simulink model "Vehicle_Model_Track_contABS"  (R2022b)
settings: Solver=ode2  StartTime=T0  StopTime=Tf  FixedStep=Ts  EnableMultiTasking=on
model workspace (MAT data in the model file):
  aKalman : Simulink.Parameter (value not decoded)
  slipEnabler : Simulink.Parameter (value not decoded)
values from neighbouring files (symbols this model uses):
  enable_onlinePlots = 0    [mainVehicleModel_2Track_contABS.m]
  enable_zoom = 1    [mainVehicleModel_2Track_contABS.m]
  hv = 0.2    [mainVehicleModel_2Track_contABS.m]
  lambda1_th = 0.1    [mainVehicleModel_2Track_contABS.m]
  lambda2_th = 0.1    [mainVehicleModel_2Track_contABS.m]
  LLC_sampleTime = LLC.sample_time    [mainVehicleModel_2Track_contABS.m]
  longCTRparam = longitController()    [mainVehicleModel_2Track_contABS.m]
  low_level_control = scenario_data.vehicle_control.low_level_control    [mainVehicleModel_2Track_contABS.m]
  omega_LPF = 100    [mainVehicleModel_2Track_contABS.m]
  previewPointParams = previewPointControllerParams()    [mainVehicleModel_2Track_contABS.m]
  rho = 0.97    [mainVehicleModel_2Track_contABS.m]
  rho_off = 0.9    [mainVehicleModel_2Track_contABS.m]
  rho_on = 1.02    [mainVehicleModel_2Track_contABS.m]
  road_data_sampled = [scenario_data.path.x_sampled', scenario_data.path.y_sampled']    [mainVehicleModel_2Track_contABS.m]
  T0 = scenario_data.times.t0    [mainVehicleModel_2Track_contABS.m]
  tau_delta = vehicle_data.steering_system.tau_D    [mainVehicleModel_2Track_contABS.m]
  Tb_dot_max = 5e3    (= 5000)    [mainVehicleModel_2Track_contABS.m]
  Tb_max = 3500    [mainVehicleModel_2Track_contABS.m]
  Tf = scenario_data.times.tf    [mainVehicleModel_2Track_contABS.m]
  Ts = scenario_data.times.step_size    [mainVehicleModel_2Track_contABS.m]
  v_on = 2.5    [mainVehicleModel_2Track_contABS.m]
  v_stop = 0.1    [mainVehicleModel_2Track_contABS.m]
  vehicle_data = getVehicleDataStruct()    [mainVehicleModel_2Track_contABS.m]
  X0 = loadInitialConditions(scenario_data.vehicle_control.max_speed/3.6)    [mainVehicleModel_2Track_contABS.m]
undefined symbols (not defined in the file or in its folder): DiscIntNeverNeededParam, latContr_select
libraries: simulink_extras x20, simulink x9, dspsigops x4, drivingvehiclecontroller x2
(part 2 of 2)

== matlab function Vehicle_Model_Track_contABS/ABS and Wheel torque generation/ABS Rear Right Wheel/compute lambda ==
  data: u input; lambda output; omega input; vehicle_data parameter
function lambda = compute_lambda(u, omega, vehicle_data)

lambda = (u - omega*vehicle_data.rear_wheel.Rr)/u;

== matlab function Vehicle_Model_Track_contABS/Vehicle Model ==
  settings: sampleTime=step_size
  data: dX_prev input; X input; Tw__rr_brake input; Tw__rl_brake input; Tw__fr_brake input; Tw__fl_brake input; Tm_req input; dX output; extra_params output; delta_req input; vehicle_data parameter; road_condition input
function [dX,extra_params] = Vehicle_model(dX_prev,X,Tw__rr_brake,Tw__rl_brake,Tw__fr_brake,Tw__fl_brake,Tm_req,delta_req,vehicle_data,road_condition)

% ----------------------------------------------------------------
%% Double Track Vehicle Model
%  authors: 
%  rev. 1.0 Mattia Piccinini & Gastone Pietro Papini Rosati
%  rev. 2.0 Edoardo Pagot
%  date:
%  rev 1.0:    13/10/2020
%  rev 2.0:    16/05/2022
% ----------------------------------------------------------------


% ----------------------------------------------------------------
%% INPUTS OF THE MODEL
% ----------------------------------------------------------------

% Model inputs are: 
%       - requested wheel torques
%       - requested steering angle at the steering wheel delta_req (in [rad])


% ----------------------------------------------------------------
%% OUTPUTS OF THE MODEL
% ----------------------------------------------------------------

% The outputs of the model are the derivatives of all vehicle states,
% collected in the dX vector, as well as some other useful extra parameters 
% to describe vehicle behavior, saved in the extra_params vector

% Empty output vectors are here initialized 
dX = zeros(23,1);  
extra_params = zeros(23,1);  


% ----------------------------------------------------------------
%% STATES OF THE MODEL
% ----------------------------------------------------------------

x         = X(1);       % [m] x-coord of the vehicle CoM
y         = X(2);       % [m] x-coord of the vehicle CoM
psi       = X(3);       % [rad] yaw angle
u         = X(4);       % [m/s] vehicle longitudinal speed
v         = X(5);       % [m/s] vehicle lateral speed
Omega     = X(6);       % [rad/s] yaw rate
Fz__rr    = X(7);       % [N] vertical force for the rear right wheel
Fz__rl    = X(8);       % [N] vertical force for the rear left wheel
Fz__fr    = X(9);       % [N] vertical force for the front right wheel
Fz__fl    = X(10);      % [N] vertical force for the front left wheel
delta     = X(11);      % [rad] steering angle (at the wheel)
omega__rr = X(12);      % [rad/s] rotational speed rear right wheel
omega__rl = X(13);      % [rad/s] rotational speed rear left wheel 
omega__fr = X(14);      % [rad/s] rotational speed front right wheel 
omega__fl = X(15);      % [rad/s] rotational speed front left wheel 
alpha__rr = X(16);      % [rad] side slip angle rear right wheel
alpha__rl = X(17);      % [rad] side slip angle rear left wheel
alpha__fr = X(18);      % [rad] side slip angle front right wheel
alpha__fl = X(19);      % [rad] side slip angle front left wheel
kappa__rr = X(20);      % [-] longitudinal slip rear right wheel
kappa__rl = X(21);      % [-] longitudinal slip rear left wheel
kappa__fr = X(22);      % [-] longitudinal slip front right wheel
kappa__fl = X(23);      % [-] longitudinal slip front left wheel

% ----------------------------------------------------------------
%% AUXILIARY MODELS
% ----------------------------------------------------------------

% ----------------------
% MOTOR MODEL
% ----------------------
% Driving torques at the wheels
Tw__rr_traction = MotorModel(Tm_req,omega__rr,vehicle_data);
Tw__rl_traction = MotorModel(Tm_req,omega__rl,vehicle_data);

% Rear wheels braking model
Tw__rr_brake = brakeModelRear(Tw__rr_brake,omega__rr,vehicle_data); 
Tw__rl_brake = brakeModelRear(Tw__rl_brake,omega__rl,vehicle_data); 
% Front wheels braking model
Tw__fr_brake = brakeModelFront(Tw__fr_brake,omega__fr,vehicle_data);
Tw__fl_brake = brakeModelFront(Tw__fl_brake,omega__fl,vehicle_data);

% Total Torques
Tw__rr = Tw__rr_brake + Tw__rr_traction;
Tw__rl = Tw__rl_brake + Tw__rl_traction;
Tw__fr = Tw__fr_brake;
Tw__fl = Tw__fl_brake;


% ----------------------
% CAMBER MODEL
% ----------------------
[gamma__rr, gamma__rl, gamma__fr, gamma__fl] = camberModel(vehicle_data);

% ----------------------
% ACKERMANN STEERING MODEL
% ----------------------
% Compute steering angles for front wheels, with perfect Ackerman steering model
[delta__fr, delta__fl] = perfectAcker(delta,vehicle_data);

% ----------------------
% AERODYNAMIC MODEL
% ----------------------
% Aero drag, downforce at rear axle, downforce at front axle
[FAxc, FAz__r, FAz__f] = aeroModel(u,vehicle_data);

% ----------------------
% LONGITUDINAL SLIPS
% ----------------------
% Longitudinal slip model including a correction for low speed 
[kappa__rr_corr,kappa__rl_corr,kappa__fr_corr,kappa__fl_corr] = long_slip_low_speed(u,Omega,kappa__rr,kappa__rl,kappa__fr,kappa__fl,omega__rr,omega__rl,omega__fr,omega__fl,delta__fr,delta__fl,Fz__rr,Fz__rl,Fz__fr,Fz__fl,gamma__rr,gamma__rl,gamma__fr,gamma__fl,vehicle_data, road_condition);
          
% ----------------------
% ROAD CONDITION
% ----------------------
% Compute the aderenace of the asphalt 
road_condition_rr = road_condition(1);
road_condition_rl = road_condition(2);
road_condition_fr = road_condition(3);
road_condition_fl = road_condition(4);

% ----------------------
% TIRE PACEJKA MODEL
% ----------------------
% Ensure symmetric behavior of left and right tires by calculating the
% forces and moments for left tires via a previous change of sign of the
% side slip alpha and the camber gamma
% Side slip sign must be changed since data were fitted with reverse alpha
% sign

% RR
Fx__rr =  MF96_FX(kappa__rr_corr, -alpha__rr, -gamma__rr, Fz__rr, vehicle_data.tyre_data_r, road_condition_rr);
Fy__rr = -MF96_FY(kappa__rr_corr,  alpha__rr, -gamma__rr, Fz__rr, vehicle_data.tyre_data_r, road_condition_rr); % mirrored
AM__rr = -MF96_MZ(kappa__rr_corr,  alpha__rr, -gamma__rr, Fz__rr, vehicle_data.tyre_data_r, road_condition_rr); % mirrored

% RL
Fx__rl = MF96_FX(kappa__rl_corr, -alpha__rl, gamma__rl, Fz__rl, vehicle_data.tyre_data_r, road_condition_rl);
Fy__rl = MF96_FY(kappa__rl_corr, -alpha__rl, gamma__rl, Fz__rl, vehicle_data.tyre_data_r, road_condition_rl);
AM__rl = MF96_MZ(kappa__rl_corr, -alpha__rl, gamma__rl, Fz__rl, vehicle_data.tyre_data_r, road_condition_rl);

%FR
Fx__fr =  MF96_FX(kappa__fr_corr, -alpha__fr, -gamma__fr, Fz__fr, vehicle_data.tyre_data_f, road_condition_fr);
Fy__fr = -MF96_FY(kappa__fr_corr,  alpha__fr, -gamma__fr, Fz__fr, vehicle_data.tyre_data_f, road_condition_fr); % mirrored
AM__fr = -MF96_MZ(kappa__fr_corr,  alpha__fr, -gamma__fr, Fz__fr, vehicle_data.tyre_data_f, road_condition_fr); % mirrored

% FL
Fx__fl = MF96_FX(kappa__fl_corr, -alpha__fl, gamma__fl, Fz__fl, vehicle_data.tyre_data_f, road_condition_fl);
Fy__fl = MF96_FY(kappa__fl_corr, -alpha__fl, gamma__fl, Fz__fl, vehicle_data.tyre_data_f, road_condition_fl);
AM__fl = MF96_MZ(kappa__fl_corr, -alpha__fl, gamma__fl, Fz__fl, vehicle_data.tyre_data_f, road_condition_fl);


Mz_tires.rr = AM__rr;  Mz_tires.rl = AM__rl;  Mz_tires.fr = AM__fr;  Mz_tires.fl = AM__fl;

% ----------------------
% VERTICAL TIRE FORCES MODEL
% ----------------------
% Compute vertical tire loads
u_dot = dX_prev(4);
VerticalForces = LoadTransferModel(Omega,u,u_dot,FAz__r,FAz__f,Mz_tires,vehicle_data);
Fz__rr__ss = VerticalForces.Fz_rr_ss;
Fz__rl__ss = VerticalForces.Fz_rl_ss;
Fz__fr__ss = VerticalForces.Fz_fr_ss;
Fz__fl__ss = VerticalForces.Fz_fl_ss;

% ----------------------
% AXLE FORCES
% ----------------------
Fx__r = Fx__rr + Fx__rl;
Fx__f = Fx__fl - sin(delta__fl)*Fy__fl + Fx__fr - sin(delta__fr)*Fy__fr;
Fy__r = Fy__rl + Fy__rr;
Fy__f = sin(delta__fl)*Fx__fl + Fy__fl + sin(delta__fr)*Fx__fr + Fy__fr;
Delta__Fx__r = (Fx__rr-Fx__rl)/2;
Delta__Fx__f = ((Fx__fr - sin(delta__fr)*Fy__fr) - (Fx__fl - sin(delta__fl)*Fy__fl))/2;


% ----------------------
% STEADY STATE SLIPS
% ----------------------
% Longitudinal Slips
[kappa__rr__ss,kappa__rl__ss,kappa__fr__ss,kappa__fl__ss] = steadyStateLongSlips(omega__rr,omega__rl,omega__fr,omega__fl,Omega,u,delta__fr,delta__fl,vehicle_data);
% Lateral Slips
[alpha__rr__ss,alpha__rl__ss,alpha__fr__ss,alpha__fl__ss] = steadyStateLatSlips(Omega,u,v,delta__fr,delta__fl,vehicle_data);


% ----------------------------------------------------------------
%% VEHICLE DATA
% ----------------------------------------------------------------
m      = vehicle_data.vehicle.m;
Lf     = vehicle_data.vehicle.Lf;
Lr     = vehicle_data.vehicle.Lr;
Wf     = vehicle_data.vehicle.Wf;
Wr     = vehicle_data.vehicle.Wr;
izz    = vehicle_data.vehicle.i_zz;
tau__N = vehicle_data.suspension.tau_N;
tau__D = vehicle_data.steering_system.tau_D;
tau__H = vehicle_data.steering_system.tau_H;
ly     = vehicle_data.vehicle.ly;
lx     = vehicle_data.vehicle.lx;
iwa__r = vehicle_data.rear_wheel.iwa_r;
iwa__f = vehicle_data.front_wheel.iwa_f;
Rr     = vehicle_data.rear_wheel.Rr;
Rf     = vehicle_data.front_wheel.Rf;

% ----------------------------------------------------------------
%% VEHICLE MODEL DIFFERENTIAL EQUATIONS
% ----------------------------------------------------------------

% The following system of ODE is imported from Maple symbolic model

% Evolution of vehicle pose
x_dot        = u*cos(psi) - v*sin(psi);
y_dot        = v*cos(psi) + u*sin(psi);
psi_dot      = Omega;
% Newton equations
u_Dot        = (Omega * m * v - FAxc + Fx__f + Fx__r) / m;
v_Dot        = (-Omega * m * u + Fy__f + Fy__r) / m;
% Euler equation
Omega_Dot    = (Lf * Fy__f - Lr * Fy__r + Wf * Delta__Fx__f + Wr * Delta__Fx__r + AM__fl + AM__fr + AM__rl + AM__rr) / izz;
% Vertical loads first order dynamics
Fz_rr_Dot    = (-Fz__rr + Fz__rr__ss) / tau__N;
Fz_rl_Dot    = (-Fz__rl + Fz__rl__ss) / tau__N;
Fz_fr_Dot    = (-Fz__fr + Fz__fr__ss) / tau__N;
Fz_fl_Dot    = (-Fz__fl + Fz__fl__ss) / tau__N;
% Steering wheel first order dynamics
delta_Dot    = (-delta * tau__D + delta_req) / tau__D / tau__H;
% Side slip angle first order dynamics
alpha_rr_Dot = -(alpha__rr - alpha__rr__ss) * abs(u) / ly;
alpha_rl_Dot = -(alpha__rl - alpha__rl__ss) * abs(u) / ly;
alpha_fr_Dot = -(alpha__fr - alpha__fr__ss) * abs(u) / ly;
alpha_fl_Dot = -(alpha__fl - alpha__fl__ss) * abs(u) / ly;
% Longitudinal slip first order dynamics
kappa_rr_Dot = -abs(u) * (kappa__rr - kappa__rr__ss) / lx;
kappa_rl_Dot = -abs(u) * (kappa__rl - kappa__rl__ss) / lx;
kappa_fr_Dot = -abs(u) * (kappa__fr - kappa__fr__ss) / lx;
kappa_fl_Dot = -abs(u) * (kappa__fl - kappa__fl__ss) / lx;
% Wheel spin dynamics
omega_rr_Dot = (-Fx__rr * Rr + Tw__rr) / iwa__r;
omega_rl_Dot = (-Fx__rl * Rr + Tw__rl) / iwa__r;
omega_fr_Dot = (-Fx__fr * Rf + Tw__fr) / iwa__f;
omega_fl_Dot = (-Fx__fl * Rf + Tw__fl) / iwa__f;

% Collect states derivatives in the dX vector
dX(1)  = x_dot;
dX(2)  = y_dot;
dX(3)  = psi_dot;
dX(4)  = u_Dot;
dX(5)  = v_Dot;
dX(6)  = Omega_Dot;
dX(7)  = Fz_rr_Dot;
dX(8)  = Fz_rl_Dot;
dX(9)  = Fz_fr_Dot;
dX(10) = Fz_fl_Dot;
dX(11) = delta_Dot;
dX(12) = omega_rr_Dot;
dX(13) = omega_rl_Dot;
dX(14) = omega_fr_Dot;
dX(15) = omega_fl_Dot;
dX(16) = alpha_rr_Dot;
dX(17) = alpha_rl_Dot;
dX(18) = alpha_fr_Dot;
dX(19) = alpha_fl_Dot;
dX(20) = kappa_rr_Dot;
dX(21) = kappa_rl_Dot;
dX(22) = kappa_fr_Dot;
dX(23) = kappa_fl_Dot;


% ----------------------------------------------------------------
%% SAVE USEFUL EXTRA PARAMETERS
% ----------------------------------------------------------------

extra_params(1)  = Tw__rr;
extra_params(2)  = Tw__rl;
extra_params(3)  = Tw__fr;
extra_params(4)  = Tw__fl;
extra_params(5)  = Fx__rr;
extra_params(6)  = Fx__rl;
extra_params(7)  = Fx__fr;
extra_params(8)  = Fx__fl;
extra_params(9)  = Fy__rr;
extra_params(10) = Fy__rl;
extra_params(11) = Fy__fr;
extra_params(12) = Fy__fl;
extra_params(13) = AM__rr;
extra_params(14) = AM__rl;
extra_params(15) = AM__fr;
extra_params(16) = AM__fl;
extra_params(17) = gamma__rr;
extra_params(18) = gamma__rl;
extra_params(19) = gamma__fr;
extra_params(20) = gamma__fl;
extra_params(21) = delta__fr;
extra_params(22) = delta__fl;
extra_params(23) = delta_req;

end

== stateflow chart Vehicle_Model_Track_contABS/ABS and Wheel torque generation/ABS Rear Left Wheel/Antilock Braking System/Activation and Deactivation Logic ==
  state abs_OFF
    ABS_ON = 0;
    state High_Speed_OFF
      Tb_select = 1;
    state Low_Speed_OFF
      Tb_select = 1;
    (default) -> High_Speed_OFF
    High_Speed_OFF -> Low_Speed_OFF [order 2] : [v < v_on - hv]
    Low_Speed_OFF -> High_Speed_OFF : [v > v_on + hv]
  state abs_ON
    ABS_ON = 1;
    state High_Speed_ON
      Tb_select = 2;
    state Low_Speed_ON
      Tb_select = 3;
    High_Speed_ON -> Low_Speed_ON [order 2] : [v < v_on]
  (default) -> abs_OFF
  High_Speed_OFF -> High_Speed_ON [order 1] : [v > v_on && ...
      | Tb_Dr > rho_on * Tb_Ctrl && ...
      | lambda > lambda1_th - (((lambda1_th - lambda2_th) * Tb_dot) / Tb_dot_max) ]
  High_Speed_ON -> High_Speed_OFF [order 1] : [Tb_Dr < rho_off * Tb_Ctrl]
  Low_Speed_ON -> Low_Speed_OFF : [v < v_stop || ...
      | Tb_Dr < rho_off * Tb_LPF]
  data: Tb_select output; Tb_Dr input; Tb_Ctrl input; v input; Tb_dot input; Tb_dot_max parameter; v_on parameter; rho_on parameter; Tb_LPF input; lambda input; lambda1_th parameter; v_stop parameter; hv parameter; rho_off parameter; ABS_ON output; lambda2_th parameter

== matlab function Vehicle_Model_Track_contABS/ABS and Wheel torque generation/ABS Rear Left Wheel/compute lambda ==
  data: u input; lambda output; omega input; vehicle_data parameter
function lambda = compute_lambda(u, omega, vehicle_data)

lambda = (u - omega*vehicle_data.rear_wheel.Rr)/u;

== stateflow chart Vehicle_Model_Track_contABS/ABS and Wheel torque generation/ABS Front Right Wheel/Antilock Braking System/Activation and Deactivation Logic ==
  state abs_OFF
    ABS_ON = 0;
    state High_Speed_OFF
      Tb_select = 1;
    state Low_Speed_OFF
      Tb_select = 1;
    (default) -> High_Speed_OFF
    High_Speed_OFF -> Low_Speed_OFF [order 2] : [v < v_on - hv]
    Low_Speed_OFF -> High_Speed_OFF : [v > v_on + hv]
  state abs_ON
    ABS_ON = 1;
    state High_Speed_ON
      Tb_select = 2;
    state Low_Speed_ON
      Tb_select = 3;
    High_Speed_ON -> Low_Speed_ON [order 2] : [v < v_on]
  (default) -> abs_OFF
  High_Speed_OFF -> High_Speed_ON [order 1] : [v > v_on && ...
      | Tb_Dr > rho_on * Tb_Ctrl && ...
      | lambda > lambda1_th - (((lambda1_th - lambda2_th) * Tb_dot) / Tb_dot_max) ]
  High_Speed_ON -> High_Speed_OFF [order 1] : [Tb_Dr < rho_off * Tb_Ctrl]
  Low_Speed_ON -> Low_Speed_OFF : [v < v_stop || ...
      | Tb_Dr < rho_off * Tb_LPF]
  data: Tb_select output; Tb_Dr input; Tb_Ctrl input; v input; Tb_dot input; Tb_dot_max parameter; v_on parameter; rho_on parameter; Tb_LPF input; lambda input; lambda1_th parameter; v_stop parameter; hv parameter; rho_off parameter; ABS_ON output; lambda2_th parameter

== matlab function Vehicle_Model_Track_contABS/ABS and Wheel torque generation/ABS Front Right Wheel/compute lambda ==
  data: u input; lambda output; omega input; vehicle_data parameter
function lambda = compute_lambda(u, omega, vehicle_data)

lambda = (u - omega*vehicle_data.rear_wheel.Rr)/u;

== stateflow chart Vehicle_Model_Track_contABS/ABS and Wheel torque generation/ABS Front Left Wheel/Antilock Braking System/Activation and Deactivation Logic ==
  state abs_OFF
    ABS_ON = 0;
    state High_Speed_OFF
      Tb_select = 1;
    state Low_Speed_OFF
      Tb_select = 1;
    (default) -> High_Speed_OFF
    High_Speed_OFF -> Low_Speed_OFF [order 2] : [v < v_on - hv]
    Low_Speed_OFF -> High_Speed_OFF : [v > v_on + hv]
  state abs_ON
    ABS_ON = 1;
    state High_Speed_ON
      Tb_select = 2;
    state Low_Speed_ON
      Tb_select = 3;
    High_Speed_ON -> Low_Speed_ON [order 2] : [v < v_on]
  (default) -> abs_OFF
  High_Speed_OFF -> High_Speed_ON [order 1] : [v > v_on && ...
      | Tb_Dr > rho_on * Tb_Ctrl && ...
      | lambda > lambda1_th - (((lambda1_th - lambda2_th) * Tb_dot) / Tb_dot_max) ]
  High_Speed_ON -> High_Speed_OFF [order 1] : [Tb_Dr < rho_off * Tb_Ctrl]
  Low_Speed_ON -> Low_Speed_OFF : [v < v_stop || ...
      | Tb_Dr < rho_off * Tb_LPF]
  data: Tb_select output; Tb_Dr input; Tb_Ctrl input; v input; Tb_dot input; Tb_dot_max parameter; v_on parameter; rho_on parameter; Tb_LPF input; lambda input; lambda1_th parameter; v_stop parameter; hv parameter; rho_off parameter; ABS_ON output; lambda2_th parameter

== matlab function Vehicle_Model_Track_contABS/Estimate pose/Online Trajectory Plots/Plot manager ==
  data: vehiclePose input; targetPoint_steerCtrl input; enable_zoomMPC input; refPath input; latContr_type input
function real_time_plot(vehiclePose,targetPoint_steerCtrl,enable_zoomMPC,refPath,latContr_type)
    
    coder.extrinsic('patch');
    
    %% Extract vehicle pose
    xCoMCar = vehiclePose(1);
    yCoMCar = vehiclePose(2);
    vehicleAttitude = vehiclePose(3);
    
    %% Load vehicle data
    vehicle_data = getVehicleDataStruct();
    Lf = vehicle_data.vehicle.Lf;        
    Lr = vehicle_data.vehicle.Lr;                 
    Wf = vehicle_data.vehicle.Wf;     
    Wr = vehicle_data.vehicle.Wr;
    
    %% Delete the plots for the previous iteration
    cla;
    
    %% Sketch the vehicle and its position, for this MPC iteration
    % Rotation matrix from vehicle (mobile) frame to the absolute frame
    RotMat = [cos(vehicleAttitude), -sin(vehicleAttitude); ...
              sin(vehicleAttitude), cos(vehicleAttitude)];
    
    pos_vehRR = RotMat*[-Lr -Wr/2]';
    pos_vehRL = RotMat*[-Lr +Wr/2]';
    pos_vehFR = RotMat*[+Lf -Wf/2]';
    pos_vehFL = RotMat*[+Lf +Wf/2]';
    pos_veh   = [pos_vehRR pos_vehRL pos_vehFL pos_vehFR];
    
    % Optimal route computed with route planner
    X_route = refPath(:,1);
    Y_route = refPath(:,2);
    plot(X_route,Y_route,'go','MarkerSize',2)
    
    % Current vehicle pose
    patch(xCoMCar + pos_veh(1,:),yCoMCar + pos_veh(2,:),'yellow');
    
    % Objects of the road scenario (walls, fixed obstacles etc)
%     for ii=1:size(mapObjects,1)
%         rectangle('Position',mapObjects(ii,:),'FaceColor',color('purple'),'EdgeColor',color('purple'),'LineWidth',2)
%     end
    
    % Target point used by some low-level lateral controllers
    if (latContr_type==1 || latContr_type==4)  
        plot(targetPoint_steerCtrl(1),targetPoint_steerCtrl(2),'r*','MarkerSize',6)
    end
    
    % Zoom on the vehicle if required
    if (enable_zoomMPC)
        xlim([xCoMCar-40 xCoMCar+40])
        ylim([yCoMCar-40 yCoMCar+40])
    end
    
end

== matlab function Vehicle_Model_Track_contABS/ABS and Wheel torque generation/ABS Front Left Wheel/compute lambda ==
  data: u input; lambda output; omega input; vehicle_data parameter
function lambda = compute_lambda(u, omega, vehicle_data)

lambda = (u - omega*vehicle_data.rear_wheel.Rr)/u;

== matlab function Vehicle_Model_Track_contABS/MATLAB Function ==
  data: start input; stop input; step input; idx input
% progress_bar is a simple utility developed to easily incorporate a progress
% bar in any MATLAB loop.
%
% Authors
% -------
%  - Sebastiano Taddei.
%
function progress_bar(start, stop, step, idx)
%PROGRESS_BAR
%   Prints a progress bar to the console.
%
%   Arguments
%   ---------
%    - start -> start index.
%    - stop  -> stop index.
%    - step  -> step to take.
%    - idx   -> current index.
%    - type  -> the type of progress bar:
%                - 0 -> XXX%;
%                - 1 -> [===    ].
%

coder.extrinsic('fprintf');

last = floor( (stop - start) / step ) * step + start;
perc = floor( idx / (last - start) * 100 );

if idx ~= start
    fprintf('\b\b\b\b\b%3d%%\n', perc);
else
    fprintf('%3d%%\n', perc);
end

end

== matlab function Vehicle_Model_Track_contABS/Driver/Lateral Controller/Preview point lateral Controller/Preview Point Controller ==
  data: target_Point input; delta output; ke input; kp input; endOfCircuit input
function delta  = previewPoint(target_Point,ke,kp,endOfCircuit)

    delta = target_Point(1) * ke + target_Point(3) * kp;
   
end

== matlab function Vehicle_Model_Track_contABS/Driver/Lateral Controller/Arc Path Following Controller/Arc Path Following Controller ==
  data: target_Point input; delta output; pose input; endOfCircuit input
function delta  = arcPathFollowController(target_Point,pose,endOfCircuit)

    % Load vehicle params
    vehicle_params = getVehicleDataStruct();
    Lf = vehicle_params.vehicle.Lf;        
    Lr = vehicle_params.vehicle.Lr;    
    L  = Lf + Lr;  % [m] vehicle wheelbase
    
    % Current vehicle center of mass pose 
    x_C     = pose(1);
    y_C     = pose(2);
    theta_C = pose(3);  % vehicle attitude (in radians)
     
    % Rotation matrix from vehicle frame to absolute frame
    Rot_mat = [cos(theta_C), -sin(theta_C); ...
               sin(theta_C),  cos(theta_C)];
    
    % Point of the vehicle in correspondence with the rear axle
    x_R = x_C - Lr*cos(theta_C);
    y_R = y_C - Lr*sin(theta_C);
    current_point = [x_R y_R];
    
    % Express the current_point in the vehicle frame
    current_point_vehFrame = [-Lr,0];
    
    % Distance from the current position to the target point
    distFromTarget = sqrt((target_Point(1)-current_point(1))^2 + (target_Point(2)-current_point(2))^2);
    
    % Express the target_Point in the vehicle frame
    target_Point_vehFrame = Rot_mat'*(target_Point(1:2)' - current_point');
    
    % Angle measured w.r.t. the vehicle reference frame
    gamma = atan2((target_Point_vehFrame(2)-current_point_vehFrame(2))/distFromTarget,(target_Point_vehFrame(1)-current_point_vehFrame(1))/distFromTarget);
    
    % Required curvature radius
    R = 0.5*distFromTarget/sin(gamma);
   
    if (~endOfCircuit)
        delta = atan(L/R);    
    else
        delta = 0;
    end

end

== matlab function Vehicle_Model_Track_contABS/ABS and Wheel torque generation/Powertrain ==
  data: ped input; vehicle_data parameter; Tw__rr_brake output; Tw__rl_brake output; Tw__fr_brake output; Tw__fl_brake output; Tm_req output
function [Tw__rr_brake,Tw__rl_brake,Tw__fr_brake,Tw__fl_brake,Tm_req] = powertrain(ped, vehicle_data)

% ----------------------
% MOTOR MODEL
% ----------------------
% Driving torques at the wheels
Tm_req = posPart(ped)*vehicle_data.motor.maxTorque;
 
% ----------------------
% BRAKE MODEL
% ----------------------
Tb_r_req = -negPart(ped)*vehicle_data.braking.totBrakeTorque*(1-vehicle_data.braking.brakeRatio);
Tb_f_req = -negPart(ped)*vehicle_data.braking.totBrakeTorque*vehicle_data.braking.brakeRatio;


% Rear wheels braking model
Tw__rr_brake = Tb_r_req; 
Tw__rl_brake = Tb_r_req; 
% Front wheels braking model
Tw__fr_brake = Tb_f_req; 
Tw__fl_brake = Tb_f_req; 


end

== matlab function Vehicle_Model_Track_contABS/Driver/Lateral Controller/Lateral Controller Stanley Dynamic/Helper Stanley Dynamic ==
  data: pose input; currPose output
function currPose = helperStanleyDyn(pose)

    currPose = [pose(1), pose(2), rad2deg(pose(3))];

end

== stateflow chart Vehicle_Model_Track_contABS/ABS and Wheel torque generation/ABS Rear Right Wheel/Antilock Braking System/Activation and Deactivation Logic ==
  state abs_OFF
    ABS_ON = 0;
    state High_Speed_OFF
      Tb_select = 1;
    state Low_Speed_OFF
      Tb_select = 1;
    (default) -> High_Speed_OFF
    High_Speed_OFF -> Low_Speed_OFF [order 2] : [v < v_on - hv]
    Low_Speed_OFF -> High_Speed_OFF : [v > v_on + hv]
  state abs_ON
    ABS_ON = 1;
    state High_Speed_ON
      Tb_select = 2;
    state Low_Speed_ON
      Tb_select = 3;
    High_Speed_ON -> Low_Speed_ON [order 2] : [v < v_on]
  (default) -> abs_OFF
  High_Speed_OFF -> High_Speed_ON [order 1] : [v > v_on && ...
      | Tb_Dr > rho_on * Tb_Ctrl && ...
      | lambda > lambda1_th - (((lambda1_th - lambda2_th) * Tb_dot) / Tb_dot_max) ]
  High_Speed_ON -> High_Speed_OFF [order 1] : [Tb_Dr < rho_off * Tb_Ctrl]
  Low_Speed_ON -> Low_Speed_OFF : [v < v_stop || ...
      | Tb_Dr < rho_off * Tb_LPF]
  data: Tb_select output; Tb_Dr input; Tb_Ctrl input; v input; Tb_dot input; Tb_dot_max parameter; v_on parameter; rho_on parameter; Tb_LPF input; lambda input; lambda1_th parameter; v_stop parameter; hv parameter; rho_off parameter; ABS_ON output; lambda2_th parameter
